simulink model "sim_v2"  (R2023b)
settings: Solver=VariableStepAuto  StartTime=0.0  StopTime=10.0  RelTol=1e-3
undefined symbols (not defined in the file): burnDuration, const_initialPosition, const_initialVelocity, deltaVDROInsertion, delvH1, DROInsertionDirection, tDROInsertion
settings Model: Creator=Prathap  LastModifiedBy=Prathap

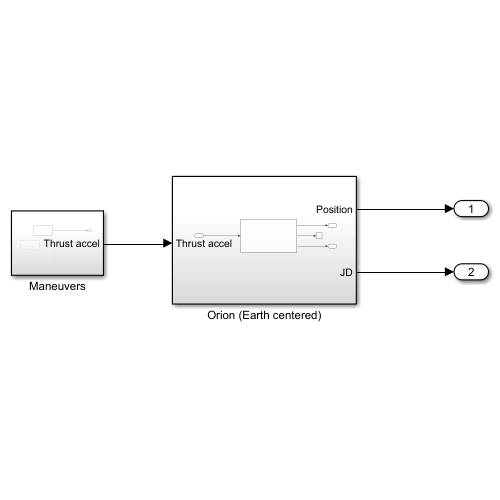
[thumbnail: Simulink's stored preview of the top-level diagram]
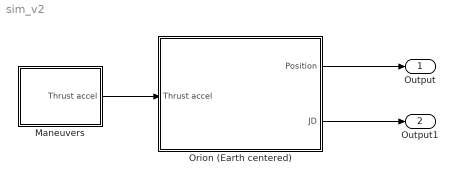
== system sim_v2 ==
  Maneuvers : Subsystem
  Orion (Earth centered) : Subsystem
  Output : Outport
  Output1 : Outport  Port=2
  wires:
  Orion (Earth centered)/2(JD) -> Output1/1
  Orion (Earth centered)/1(Position) -> Output/1
  Maneuvers/1(Thrust accel) -> Orion (Earth centered)/1(Thrust accel)

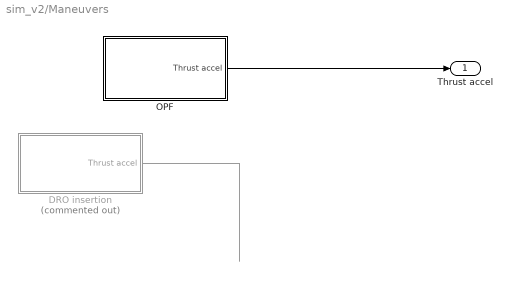
== system sim_v2/Maneuvers ==
  DRO insertion : Subsystem  Commented=on
  OPF : Subsystem
  Thrust accel : Outport
  wires:
  OPF/1(Thrust accel) -> Thrust accel/1
  DRO insertion/1(Thrust accel) -> ?

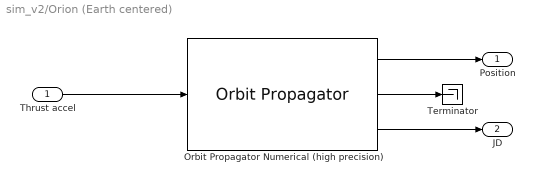
== system sim_v2/Orion (Earth centered) ==
  Thrust accel : Inport
  Orbit Propagator Numerical (high precision) : OrbitPropagator  propagator=Numerical (high precision)  accelIn=on  startDate=jd  action=None  stateFormatNum=ICRF state vector  eccentricity=0  inclination=30  raan=0  argPeriapsis=0  trueAnomaly=0  inertialPosition=const_initialPosition(:,2)  inertialVelocity=const_initialVelocity(:,2)  fixedPosition=[-4142689.0 -2676864.7 -4669861.6]  fixedVelocity=[1452.7 -6720.7 2568.1]  gravityModel=Point-mass  customR=3396200  customMu=4.305e13  customJ2=1.0826269e-03  customOmega=4.06125949e-3  useEOPs=off
  Terminator : Terminator
  Position : Outport
  JD : Outport  Port=2
  wires:
  Orbit Propagator Numerical (high precision)/1 -> Position/1
  Orbit Propagator Numerical (high precision)/2 -> Terminator/1
  Thrust accel/1 -> Orbit Propagator Numerical (high precision)/1
  Orbit Propagator Numerical (high precision)/3 -> JD/1

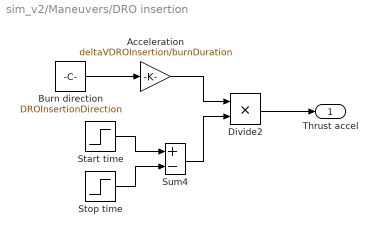
== system sim_v2/Maneuvers/DRO insertion ==
  Acceleration : Gain  Gain=deltaVDROInsertion/burnDuration
  Burn direction : Constant  Value=DROInsertionDirection
  Divide2 : Product  Inputs=**
  Start time : Step  Time=tDROInsertion  SampleTime=0
  Stop time : Step  Time=tDROInsertion+burnDuration  SampleTime=0
  Sum4 : Sum  Inputs=+-
  Thrust accel : Outport
  wires:
  Acceleration/1 -> Divide2/1
  Start time/1 -> Sum4/1
  Divide2/1 -> Thrust accel/1
  Stop time/1 -> Sum4/2
  Sum4/1 -> Divide2/2
  Burn direction/1 -> Acceleration/1

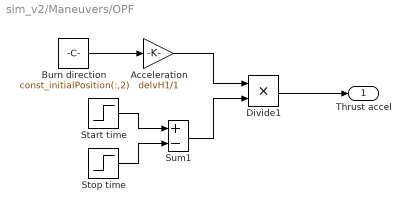
== system sim_v2/Maneuvers/OPF ==
  Acceleration : Gain  Gain=delvH1/1
  Burn direction : Constant  Value=const_initialPosition(:,2)
  Divide1 : Product  Inputs=**
  Start time : Step  Time=15060  SampleTime=0
  Stop time : Step  Time=15061  SampleTime=0
  Sum1 : Sum  Inputs=+-
  Thrust accel : Outport
  wires:
  Burn direction/1 -> Acceleration/1
  Sum1/1 -> Divide1/2
  Divide1/1 -> Thrust accel/1
  Acceleration/1 -> Divide1/1
  Start time/1 -> Sum1/1
  Stop time/1 -> Sum1/2
